simulink model "Project5_Trial"  (R2021b)
settings: Solver=VariableStepAuto  StartTime=0.0  StopTime=Sim_TIME  RelTol=1e-3
values from neighbouring files (symbols this model uses):
  Cn = 2.3*3600    (= 8280)    [Project5_Run_Trial.m]
  I = 2.3    [Project5_Run_Trial.m]
  OCV = Data(:, 2)    [Project5_Run_Trial.m]
  R_Charge = Data(:, 3)    [Project5_Run_Trial.m]
  R_Discharge = Data(:, 4)    [Project5_Run_Trial.m]
  SOC = Data(:, 1)    [Project5_Run_Trial.m]
settings Model: Creator=rohitkharat  LastModifiedBy=rohitkharat

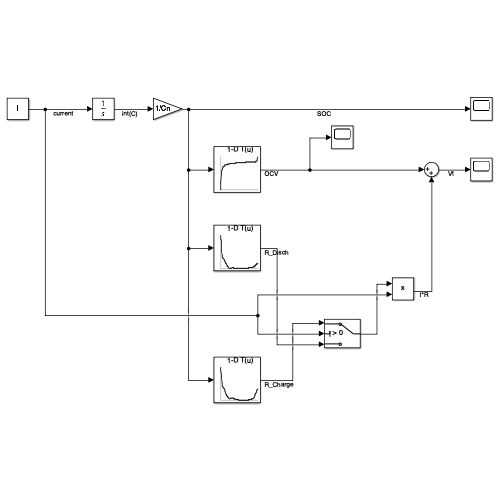
[thumbnail: Simulink's stored preview of the top-level diagram]
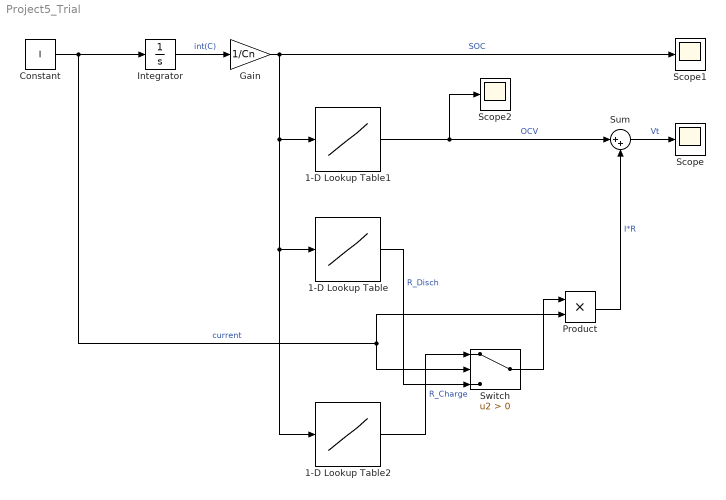
== system Project5_Trial ==
  1-D Lookup Table : Lookup_n-D  NumberOfTableDimensions=1  BreakpointsForDimension1=SOC  Table=R_Discharge  InternalRulePriority=Speed  RndMeth=Simplest  InputSameDT=on
  1-D Lookup Table1 : Lookup_n-D  NumberOfTableDimensions=1  BreakpointsForDimension1=SOC  Table=OCV  InternalRulePriority=Speed  RndMeth=Simplest  InputSameDT=on
  1-D Lookup Table2 : Lookup_n-D  NumberOfTableDimensions=1  BreakpointsForDimension1=SOC  Table=R_Charge  InternalRulePriority=Speed  RndMeth=Simplest  InputSameDT=on
  Constant : Constant  Value=I
  Gain : Gain  Gain=1/Cn
  Integrator : Integrator
  Product : Product
  Scope : Scope
  Scope1 : Scope
  Scope2 : Scope
  Sum : Sum  Inputs=|++
  Switch : Switch  Criteria=u2 > Threshold
  wires:
  Constant/1 -> Product/2, Switch/2, Integrator/1  "current"
  Integrator/1 -> Gain/1  "int(C)"
  Gain/1 -> Scope1/1, 1-D Lookup Table1/1, 1-D Lookup Table2/1, 1-D Lookup Table/1  "SOC"
  1-D Lookup Table1/1 -> Scope2/1, Sum/1  "OCV"
  1-D Lookup Table/1 -> Switch/3  "R_Disch"
  Product/1 -> Sum/2  "I*R"
  Sum/1 -> Scope/1  "Vt"
  1-D Lookup Table2/1 -> Switch/1  "R_Charge"
  Switch/1 -> Product/1
